simulink model "pendule_inv_etu"  (R2017a)
settings: Solver=VariableStepAuto  StartTime=0.0  StopTime=tf  RelTol=1e-3
values from neighbouring files (symbols this model uses):
  K = [10 1]    [exemple_test_pendule_inv_capteur.m]    (also in exemple_test_pendule_inv_echant.m = [30 10])
  ue = 0    [exemple_test_pendule_inv_capteur.m]    (also in exemple_test_pendule_inv_echant.m)
  x0 = [pi/20 0]    [exemple_test_pendule_inv_capteur.m]    (also in exemple_test_pendule_inv_echant.m)
  xe = [0 0]    [exemple_test_pendule_inv_capteur.m]    (also in exemple_test_pendule_inv_echant.m)
settings Model: Creator=jky  LastModifiedBy=jky

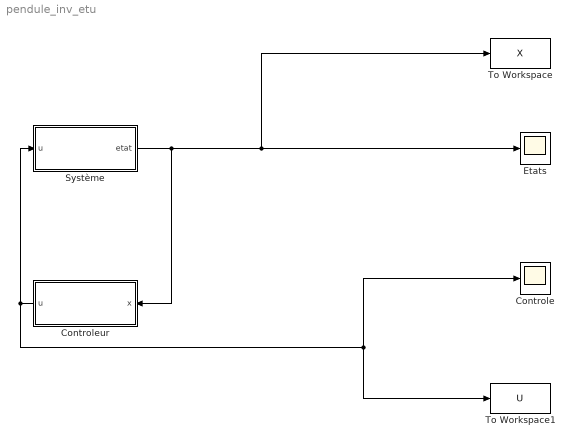
== system pendule_inv_etu ==
  Controle : Scope
  Controleur : Subsystem
  Etats : Scope
  Système : Subsystem
  To Workspace : ToWorkspace  VariableName=X  SaveFormat=Timeseries  SampleTime=-1
  To Workspace1 : ToWorkspace  VariableName=U  SaveFormat=Timeseries  SampleTime=-1
  wires:
  Système/1(etat) -> Controleur/1(x), To Workspace/1, Etats/1
  Controleur/1(u) -> To Workspace1/1, Controle/1, Système/1(u)

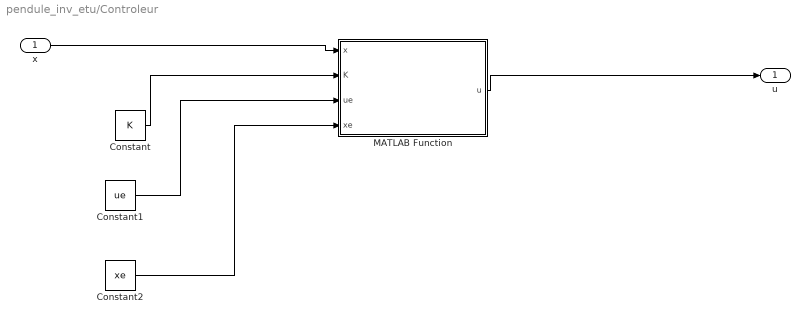
== system pendule_inv_etu/Controleur ==
  x : Inport
  Constant : Constant  Value=K
  Constant1 : Constant  Value=ue
  Constant2 : Constant  Value=xe
  MATLAB Function : MATLAB Function  TreatAsAtomicUnit=on
  u : Outport
  wires:
  x/1 -> MATLAB Function/1(x)
  MATLAB Function/1(u) -> u/1
  Constant/1 -> MATLAB Function/2(K)
  Constant1/1 -> MATLAB Function/3(ue)
  Constant2/1 -> MATLAB Function/4(xe)

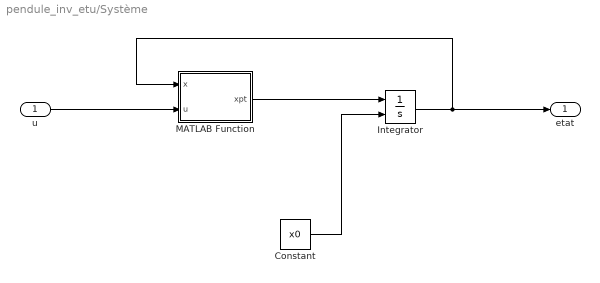
== system pendule_inv_etu/Système ==
  u : Inport
  Constant : Constant  Value=x0
  Integrator : Integrator  InitialConditionSource=external  InitialCondition=[pi/20 0]
  MATLAB Function : MATLAB Function  TreatAsAtomicUnit=on
  etat : Outport
  wires:
  u/1 -> MATLAB Function/2(u)
  Integrator/1 -> etat/1, MATLAB Function/1(x)
  MATLAB Function/1(xpt) -> Integrator/1
  Constant/1 -> Integrator/2

== matlab function pendule_inv_etu/Controleur/MATLAB Function ==
  data: x input; u output; K input; ue input; xe input
function u = fcn(x, K, ue, xe)
u = ue + transpose(K)*(x-xe);

== matlab function pendule_inv_etu/Système/MATLAB Function ==
  data: x input; u input; xpt output
function xpt = fcn(x,u)
g = 9.81;
l = 10;
xpt = transpose([x(2) ((g/l)*sin(x(1)))-((cos(x(1))*u)/l)]);
